simulink model "Finish"  (R2021b)
settings: Solver=VariableStepAuto  StartTime=0.0  StopTime=1  RelTol=1e-6
libraries: spsTriangleGeneratorLib x1
settings Model: Creator=Selected  LastModifiedBy=Selected

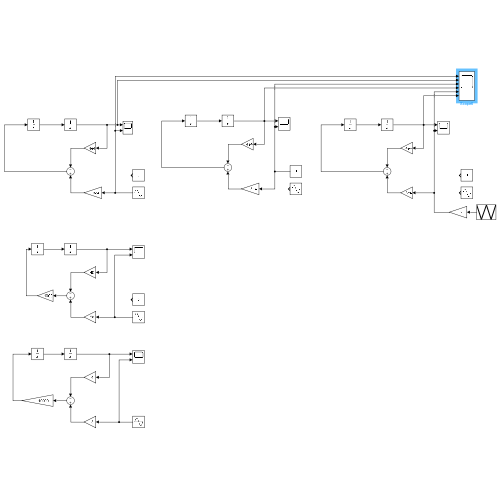
[thumbnail: Simulink's stored preview of the top-level diagram]
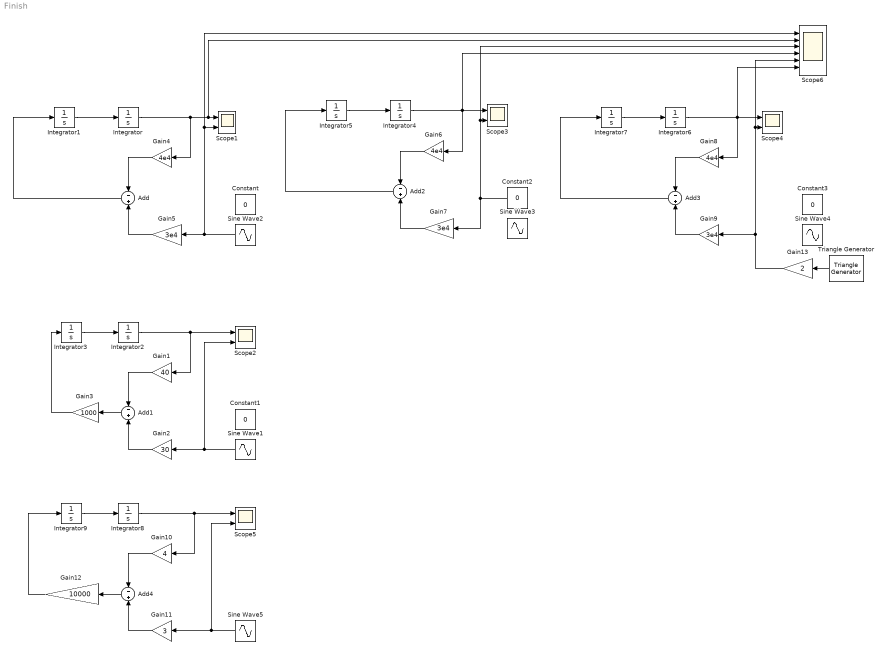
== system Finish ==
  Add{,1..4} (5 alike) : Sum  Inputs=-+
  Constant{,1..3} (4 alike) : Constant  Value=0
  Gain1 : Gain  Gain=40
  Gain10 : Gain  Gain=4
  Gain11 : Gain  Gain=3
  Gain12 : Gain  Gain=10000
  Gain13 : Gain  Gain=2
  Gain2 : Gain  Gain=30
  Gain3 : Gain  Gain=1000
  Gain4 : Gain  Gain=4e4
  Gain5 : Gain  Gain=3e4
  Gain6 : Gain  Gain=4e4
  Gain7 : Gain  Gain=3e4
  Gain8 : Gain  Gain=4e4
  Gain9 : Gain  Gain=3e4
  Integrator{,2,4,6,8} (5 alike) : Integrator  InitialCondition=1
  Integrator{1,3,5,7,9} (5 alike) : Integrator
  Scope{1..5} (5 alike) : Scope  NumInputPorts=2
  Scope6 : Scope  NumInputPorts=6
  Sine Wave1 : Sin  Amplitude=2  Frequency=95.49  SampleTime=0
  Sine Wave2 : Sin  Amplitude=2  Frequency=600  SampleTime=0
  Sine Wave3 : Sin  Amplitude=2  Frequency=600  SampleTime=0
  Sine Wave4 : Sin  Amplitude=2  Frequency=600  SampleTime=0
  Sine Wave5 : Sin  Amplitude=3  Frequency=95.49  SampleTime=0
  Triangle Generator : spsTriangleGeneratorLib/Triangle Generator  Freq=95.49  Phase=0  Ts=0
  wires:
  Integrator/1 -> Gain4/1, Scope6/2, Scope1/1
  Integrator1/1 -> Integrator/1
  Gain4/1 -> Add/1
  Gain5/1 -> Add/2
  Add/1 -> Integrator1/1
  Gain1/1 -> Add1/1
  Integrator3/1 -> Integrator2/1
  Integrator2/1 -> Gain1/1, Scope2/1
  Sine Wave1/1 -> Scope2/2, Gain2/1
  Gain2/1 -> Add1/2
  Add1/1 -> Gain3/1
  Gain3/1 -> Integrator3/1
  Gain6/1 -> Add2/1
  Integrator5/1 -> Integrator4/1
  Integrator4/1 -> Scope6/4, Gain6/1, Scope3/1
  Gain7/1 -> Add2/2
  Constant2/1 -> Gain7/1, Scope6/3, Scope3/2
  Gain8/1 -> Add3/1
  Add3/1 -> Integrator7/1
  Integrator6/1 -> Scope6/6, Scope4/1, Gain8/1
  Gain9/1 -> Add3/2
  Integrator7/1 -> Integrator6/1
  Sine Wave2/1 -> Scope6/1, Scope1/2, Gain5/1
  Gain12/1 -> Integrator9/1
  Add4/1 -> Gain12/1
  Gain11/1 -> Add4/2
  Sine Wave5/1 -> Scope5/2, Gain11/1
  Gain10/1 -> Add4/1
  Integrator9/1 -> Integrator8/1
  Add2/1 -> Integrator5/1
  Integrator8/1 -> Gain10/1, Scope5/1
  Triangle Generator/1 -> Gain13/1
  Gain13/1 -> Scope6/5, Scope4/2, Gain9/1
